simulink model "debounceNoActions"  (R2017b)
settings: Solver=FixedStepDiscrete  StartTime=0.0  StopTime=10.0  RelTol=1e-3  EnableMultiTasking=on
Description:
  | Property Proving with an Assumption Block
  | 
  | This example shows how to perform a Simulink Design Verifier property proof using a
  | Proof Assumption block.
settings Model: Creator=The MathWorks, Inc.  LastModifiedBy=hbourbou
settings SolverCC: InsertRTBMode=Auto
settings DataIOCC: LimitDataPoints=on  SaveFormat=Structure
settings OptimizationCC: DefaultParameterBehavior=Inlined  ExpressionDepthLimit=2147483647  InitFltsAndDblsToZero=on  EfficientMapNaN2IntZero=off  LifeSpan=inf
settings DebuggingCC: SaveWithParameterizedLinksMsg=none  UnderspecifiedInitializationDetection=Classic  MergeDetectMultiDrivingBlocksExec=none  SignalResolutionControl=TryResolveAllWithWarning  SolverPrmCheckMsg=warning  FcnCallInpInsideContextMsg=warning  StateNameClashWarn=warning  StrictBusMsg=Warning  SFUnexpectedBacktrackingDiag=warning  SFNoUnconditionalDefaultTransitionDiag=warning  SFExecutionAtInitializationDiag=none
settings HardwareCC: ProdBitPerPointer=32  ProdBitPerSizeT=32  ProdBitPerPtrDiffT=32  ProdLargestAtomicFloat=None  ProdIntDivRoundTo=Undefined  ProdEndianess=Unspecified  ProdWordSize=32  ProdHWDeviceType=32-bit Generic
settings ModelReferenceCC: PropagateSignalLabelsOutOfModel=off
settings SFSimCC: SimParseCustomCode=off
settings CodeAppCC: StateflowObjectComments=on
settings GRTTargetCC: TargetFcnLib=ansi_tfl_tmw.mat  TargetLangStandard=C89/C90 (ANSI)  GeneratePreprocessorConditionals=Disable all  CombineOutputUpdateFcns=off  GRTInterface=on
settings ConfigComp: DVMode=PropertyProving  DVMaxProcessTime=60  DVMakeOutputFilesUnique=off  DVParameters=on  DVModelCoverageObjectives=MCDC  DVMaxTestCaseSteps=500  DVTestSuiteOptimization=CombinedObjectives  DVAssertions=EnableAll  DVProofAssumptions=EnableAll  DVDetectActiveLogic=on  DVDetectFloatOverflow=off  DVProvingStrategy=FindViolation  DVModelReferenceHarness=on

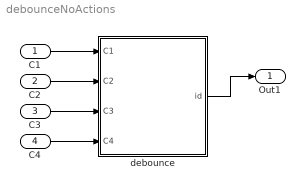
== system debounceNoActions ==
  C1 : Inport  OutDataTypeStr=boolean
  C2 : Inport  Port=2  OutDataTypeStr=boolean
  C3 : Inport  Port=3  OutDataTypeStr=boolean
  C4 : Inport  Port=4  OutDataTypeStr=boolean
  debounce : Stateflow chart  TreatAsAtomicUnit=on
  Out1 : Outport
  wires:
  debounce/1(id) -> Out1/1
  C1/1 -> debounce/1(C1)
  C2/1 -> debounce/2(C2)
  C3/1 -> debounce/3(C3)
  C4/1 -> debounce/4(C4)

== stateflow chart debounceNoActions/debounce ==
  settings: updateMethod=DISCRETE
  state To
    state To_on
      en: id = 2;
    state To_off
      en: id = 3;
  state Off
    en: id = 1;
  state OnParent
    state On
      en:  id = 4;
  (default) -> Off
  To_on -> On [order 2] : [C4]
  Off -> To_on : [C1]
  To_on -> Off [order 1] : [C2]
  To_off -> Off [order 2] : [C3]
  On -> To_off : [C1]
  To_off -> On [order 1] : [C2]
  data: id output double; C1 input boolean; C2 input boolean; C3 input boolean; C4 input boolean
